simulink subsystem "overflowing_counter"  (R2022b)
settings: Solver=VariableStepAuto  StartTime=0.0  StopTime=10.0  RelTol=1e-3
model mask{Td=1, Overflow_point=255, Increment=1}
  mask prompts: Td "Update rate"; Overflow_point "Overflow point"; Increment "Increment Rate"
settings Model: Creator=papaveneti  LastModifiedBy=papaveneti

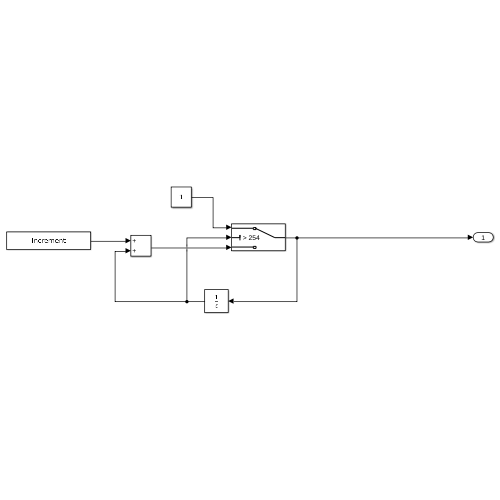
[thumbnail: Simulink's stored preview of the top-level diagram]
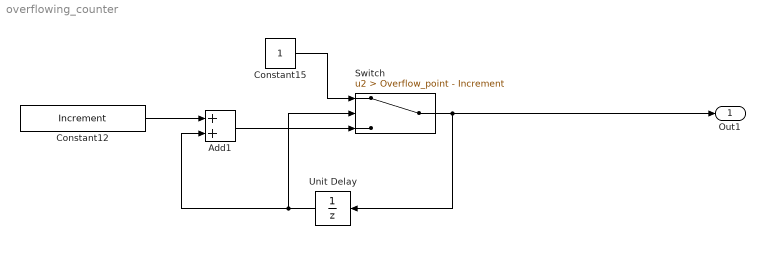
== system overflowing_counter ==
  Add1 : Sum
  Constant12 : Constant  Value=Increment
  Constant15 : Constant
  Switch : Switch  Criteria=u2 > Threshold  Threshold=Overflow_point - Increment  SaturateOnIntegerOverflow=off  InputSameDT=off
  Unit Delay : UnitDelay  InitialCondition=1-Increment  SampleTime=Td  HasFrameUpgradeWarning=on
  Out1 : Outport
  wires:
  Constant15/1 -> Switch/1
  Add1/1 -> Switch/3
  Unit Delay/1 -> Switch/2, Add1/2
  Switch/1 -> Unit Delay/1, Out1/1
  Constant12/1 -> Add1/1
